simulink model "vvvf"  (R2023a)
settings: Solver=ode23  StartTime=0.0  StopTime=6  MaxStep=5e-6  RelTol=1e-3
libraries: spsIGBTDiodeLib x6, spsAsynchronousMachineSIUnitsLib x1, spsTriangleGeneratorLib x1, spsDCVoltageSourceLib x1, spsVoltageMeasurementLib x1, sps_lib x1
settings Model: Creator=搬砖工卢卡斯  LastModifiedBy=搬砖工卢卡斯

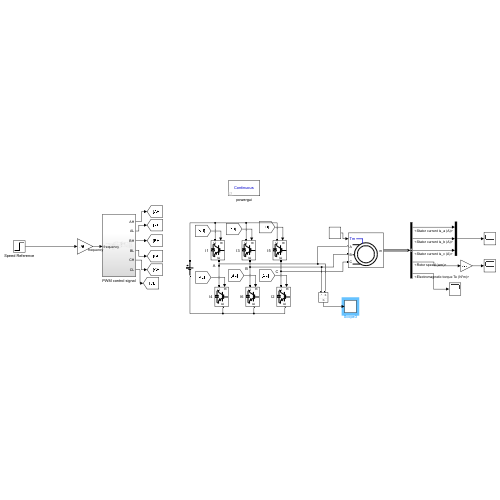
[thumbnail: Simulink's stored preview of the top-level diagram]
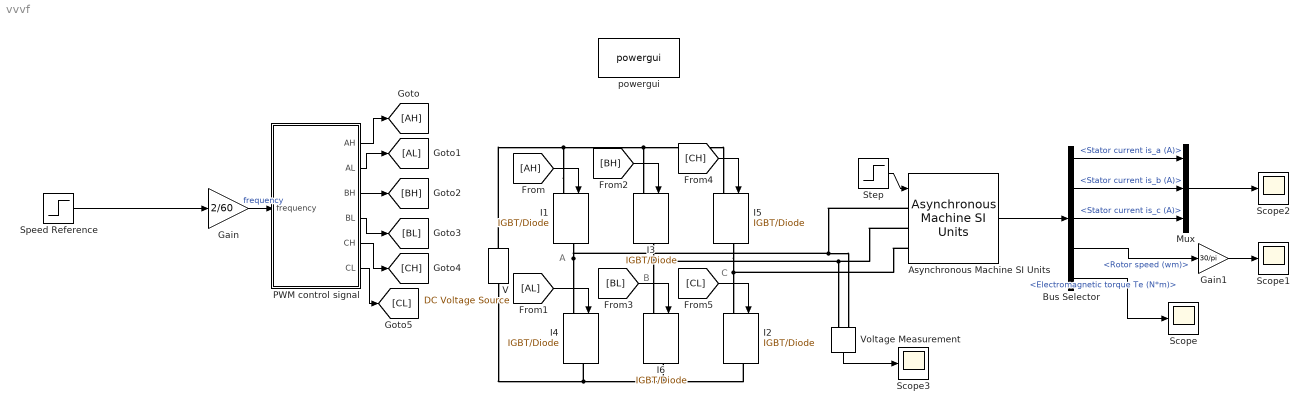
== system vvvf ==
  note: B
  note: C
  note: A
  Asynchronous Machine SI Units : spsAsynchronousMachineSIUnitsLib/Asynchronous Machine SI Units  RotorType=Squirrel-cage  PresetModel=No  MechanicalLoad=Torque Tm  ShowDetailedParameters=on  ReferenceFrame=Rotor  Units=SI  MeasurementBus=off  NominalParameters=[2200 200 50]  VoltageRatio=1  Stator=[0.877 0.0046]  Rotor=[1.47 0.0046]  Cage1=[0.4155 0.002066]  Cage2=[0.4168 0.0003495]  Lm=0.1608  Mechanical=[0.015 0 2]  PolePairs=2  InitialConditions=[1 0 0 0 0 0 0 0]  SimulateSaturation=off  Saturation=[14.03593122, 27.81365428, 53.79336849, 72.68890987, 97.98006896, 148.6815601, 215.7428561, 302.9841135, 428.7778367 ; 230, 322, 414, 460, 506, 552, 598, 644, 690]  LoadFlowParameters=1492000  TsPowergui=0  TsBlock=-1  IterativeModel=Trapezoidal non iterative  IterativeDiscreteModel=Trapezoidal non iterative  Pmec=1.492e+006
  Bus Selector : BusSelector  OutputSignals=Stator measurements.Stator current is_a (A),Stator measurements.Stator current is_b (A),Stator measurements.Stator current is_c (A),Mechanical.Rotor speed (wm),Mechanical.Electromagnetic torque Te (N*m)
  Gain : Gain  Gain=2/60
  Gain1 : Gain  Gain=30/pi
  I{1..6} (6 alike) : spsIGBTDiodeLib/IGBT//Diode  Ron=1e-3  Rs=1e5  Cs=inf  Measurements=off
  Mux : Mux  Inputs=3
  PWM control signal : Subsystem
  Scope{,1..3} (4 alike) : Scope
  Speed Reference : Step  Time=0  After=1500  SampleTime=0
  Step : Step  Time=3  After=0  SampleTime=0
  V : spsDCVoltageSourceLib/DC Voltage Source  Amplitude=500  Measurements=None
  Voltage Measurement : spsVoltageMeasurementLib/Voltage Measurement  PhasorSimulation=off  OutputType=Complex  PSBequivalent=0
  powergui : sps_lib/powergui  Priority=1  SimulationMode=Continuous  SampleTime=1e-5  frequency=60  Iterations=50  frequencyindice=50  Pbase=100e6  ErrMax=1e-4  UnitsV=kV  UnitsW=MW  buscounter=0  FunctionMessages=off  echomessages=off  EnableUseOfTLC=off  CurrentSourceSwitches=off  DisableSnubberDevices=off  DisableRonSwitches=off  DisableVfSwitches=off  DisplayEquations=off  AutomaticDiscreteSolvers=off  SolverType=Tustin/Backward Euler (TBE)  Interpol=off  ExternalGateDelay=off  methode=off  Ts=100  x0status=blocks  SPID=on  SwTol=0  HookPort=off  NonlinearTolerance=1e-4  nMaxIteration=100  ContinueOnMaxIteration=off  RestoreLinks=warning  ResistiveCurrentMeasurement=off  Frange=[0:2:500]  Ylog=off  Xlog=on  ShowGrid=off  save=off  variable=ZData  structure=0  ZoomFFT=off  StartTime=0.0  cycles=1  DisplayStyle=1  fundamental=60  FreqAxis=off  MaxFrequency=1000  frequencyindicesteady=1  RmsSteady=1  display=off
  wires:
  Speed Reference/1 -> Gain/1
  Gain/1 -> PWM control signal/1(frequency)  "frequency"
  PWM control signal/1(AH) -> [AH]
  PWM control signal/6(CL) -> [CL]
  PWM control signal/4(BL) -> [BL]
  PWM control signal/5(CH) -> [CH]
  PWM control signal/3(BH) -> [BH]
  PWM control signal/2(AL) -> [AL]
  [CH] -> I5/1
  [AH] -> I1/1
  [BH] -> I3/1
  [CL] -> I2/1
  [BL] -> I6/1
  [AL] -> I4/1
  Step/1 -> Asynchronous Machine SI Units/1
  Asynchronous Machine SI Units/1 -> Bus Selector/1
  Bus Selector/5 -> Scope/1  "<Electromagnetic torque Te (N*m)>"
  Bus Selector/4 -> Gain1/1  "<Rotor speed (wm)>"
  Gain1/1 -> Scope1/1
  Mux/1 -> Scope2/1
  Bus Selector/1 -> Mux/1  "<Stator current is_a (A)>"
  Bus Selector/2 -> Mux/2  "<Stator current is_b (A)>"
  Bus Selector/3 -> Mux/3  "<Stator current is_c (A)>"
  Voltage Measurement/1 -> Scope3/1
  connections:
  I1/RConn1 -- Asynchronous Machine SI Units/LConn1 -- Voltage Measurement/LConn1 -- I4/LConn1
  I6/RConn1 -- V/LConn1 -- I4/RConn1 -- I2/RConn1
  I1/LConn1 -- V/RConn1 -- I5/LConn1 -- I3/LConn1
  I5/RConn1 -- Asynchronous Machine SI Units/LConn3 -- I2/LConn1
  I3/RConn1 -- Asynchronous Machine SI Units/LConn2 -- Voltage Measurement/LConn2 -- I6/LConn1

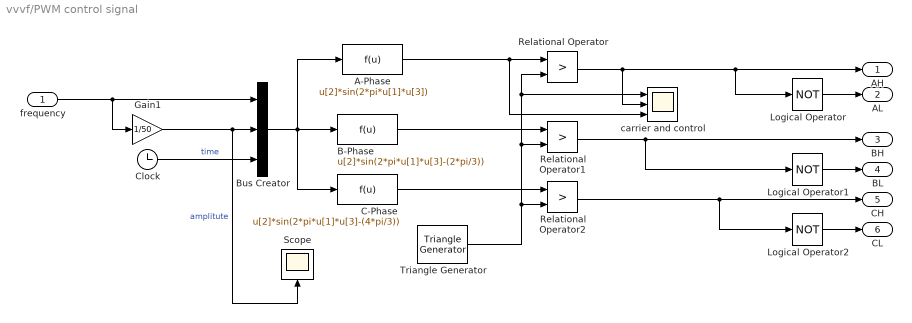
== system vvvf/PWM control signal ==
  frequency : Inport
  A-Phase : Fcn  Expr=u[2]*sin(2*pi*u[1]*u[3])
  B-Phase : Fcn  Expr=u[2]*sin(2*pi*u[1]*u[3]-(2*pi/3))
  Bus Creator : BusCreator  Inputs=3
  C-Phase : Fcn  Expr=u[2]*sin(2*pi*u[1]*u[3]-(4*pi/3))
  Clock : Clock
  Gain1 : Gain  Gain=1/50
  Logical Operator : Logic  Operator=NOT  IconShape=distinctive  AllPortsSameDT=off  OutDataTypeStr=boolean
  Logical Operator1 : Logic  Operator=NOT  IconShape=distinctive  AllPortsSameDT=off  OutDataTypeStr=boolean
  Logical Operator2 : Logic  Operator=NOT  IconShape=distinctive  AllPortsSameDT=off  OutDataTypeStr=boolean
  Relational Operator : RelationalOperator  Operator=>  OutDataTypeStr=boolean  InputSameDT=off
  Relational Operator1 : RelationalOperator  Operator=>  OutDataTypeStr=boolean  InputSameDT=off
  Relational Operator2 : RelationalOperator  Operator=>  OutDataTypeStr=boolean  InputSameDT=off
  Scope : Scope
  Triangle Generator : spsTriangleGeneratorLib/Triangle Generator  Freq=1000  Phase=90  Ts=0
  carrier and control : Scope  NumInputPorts=3
  AH : Outport
  AL : Outport  Port=2
  BH : Outport  Port=3
  BL : Outport  Port=4
  CH : Outport  Port=5
  CL : Outport  Port=6
  wires:
  frequency/1 -> Gain1/1, Bus Creator/1
  Relational Operator2/1 -> CH/1, Logical Operator2/1
  Bus Creator/1 -> C-Phase/1, B-Phase/1, A-Phase/1
  Relational Operator1/1 -> Logical Operator1/1, BH/1
  A-Phase/1 -> carrier and control/3, Relational Operator/1
  Relational Operator/1 -> carrier and control/2, AH/1, Logical Operator/1
  Triangle Generator/1 -> Relational Operator2/2, Relational Operator1/2, Relational Operator/2, carrier and control/1
  Clock/1 -> Bus Creator/3  "time"
  Gain1/1 -> Scope/1, Bus Creator/2  "amplitute"
  Logical Operator2/1 -> CL/1
  C-Phase/1 -> Relational Operator2/1
  Logical Operator/1 -> AL/1
  B-Phase/1 -> Relational Operator1/1
  Logical Operator1/1 -> BL/1
